simulink model "DUC"  (R2017b)
settings: Solver=VariableStepAuto  StartTime=0.0  StopTime=10.0  RelTol=1e-3
libraries: dspsigops x16, simulink x8
(part 2 of 2)

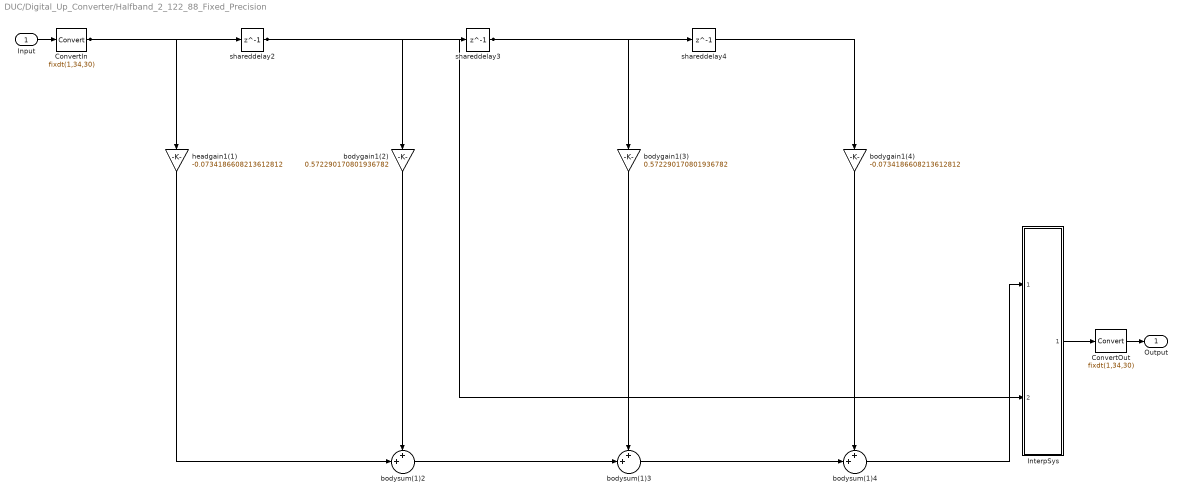
== system DUC/Digital_Up_Converter/Halfband_2_122_88_Fixed_Precision ==
  Input : Inport
  ConvertIn : DataTypeConversion  OutDataTypeStr=fixdt(1,34,30)  RndMeth=Nearest  SaturateOnIntegerOverflow=on
  ConvertOut : DataTypeConversion  OutDataTypeStr=fixdt(1,34,30)  SaturateOnIntegerOverflow=on
  InterpSys : Subsystem  Tag=FilterWizardInterpolatorCommutator
  bodygain1(2) : Gain  Gain=0.572290170801936782  ParamDataTypeStr=fixdt(1,36,34)  OutDataTypeStr=fixdt(1,36,32)  SaturateOnIntegerOverflow=on
  bodygain1(3) : Gain  Gain=0.572290170801936782  ParamDataTypeStr=fixdt(1,36,34)  OutDataTypeStr=fixdt(1,36,32)  SaturateOnIntegerOverflow=on
  bodygain1(4) : Gain  Gain=-0.0734186608213612812  ParamDataTypeStr=fixdt(1,36,34)  OutDataTypeStr=fixdt(1,36,32)  SaturateOnIntegerOverflow=on
  bodysum(1)2 : Sum  Inputs=++|  AccumDataTypeStr=fixdt(1,69,64)  OutDataTypeStr=fixdt(1,36,32)  SaturateOnIntegerOverflow=on
  bodysum(1)3 : Sum  Inputs=++|  AccumDataTypeStr=fixdt(1,69,64)  OutDataTypeStr=fixdt(1,36,32)  SaturateOnIntegerOverflow=on
  bodysum(1)4 : Sum  Inputs=++|  AccumDataTypeStr=fixdt(1,69,64)  OutDataTypeStr=fixdt(1,36,32)  SaturateOnIntegerOverflow=on
  headgain1(1) : Gain  Gain=-0.0734186608213612812  ParamDataTypeStr=fixdt(1,36,34)  OutDataTypeStr=fixdt(1,36,32)  SaturateOnIntegerOverflow=on
  shareddelay2 : Delay  DelayLength=1  InitialCondition=0
  shareddelay3 : Delay  DelayLength=1  InitialCondition=0
  shareddelay4 : Delay  DelayLength=1  InitialCondition=0
  Output : Outport
  wires:
  headgain1(1)/1 -> bodysum(1)2/2
  Input/1 -> ConvertIn/1
  ConvertIn/1 -> headgain1(1)/1, shareddelay2/1
  bodygain1(2)/1 -> bodysum(1)2/1
  bodysum(1)2/1 -> bodysum(1)3/2
  shareddelay2/1 -> bodygain1(2)/1, InterpSys/2(input2), shareddelay3/1
  bodygain1(3)/1 -> bodysum(1)3/1
  bodysum(1)3/1 -> bodysum(1)4/2
  shareddelay3/1 -> bodygain1(3)/1, shareddelay4/1
  bodygain1(4)/1 -> bodysum(1)4/1
  bodysum(1)4/1 -> InterpSys/1(input1)
  shareddelay4/1 -> bodygain1(4)/1
  InterpSys/1(output) -> ConvertOut/1
  ConvertOut/1 -> Output/1

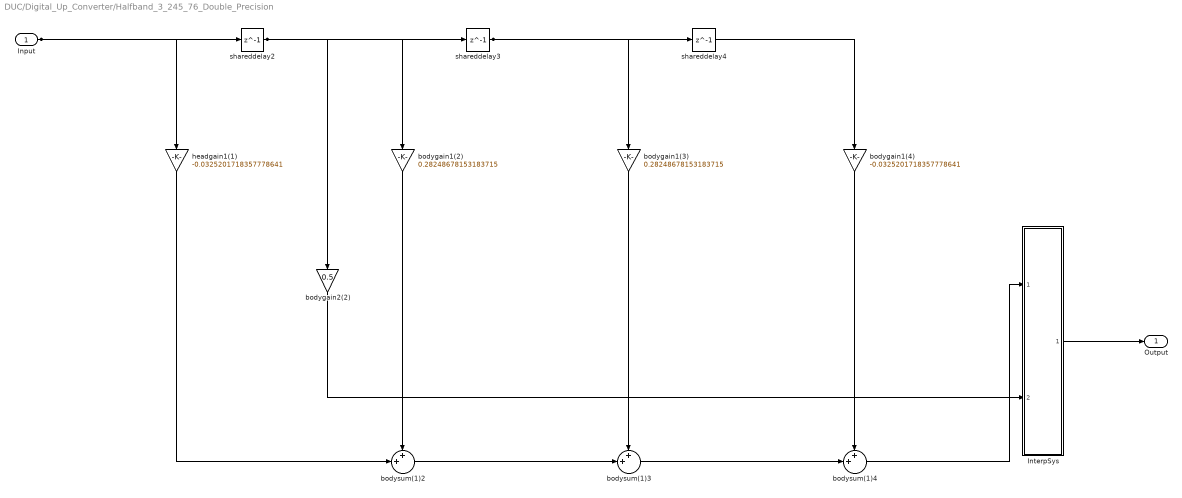
== system DUC/Digital_Up_Converter/Halfband_3_245_76_Double_Precision ==
  Input : Inport
  InterpSys : Subsystem  Tag=FilterWizardInterpolatorCommutator
  bodygain1(2) : Gain  Gain=0.28248678153183715  ParamDataTypeStr=double  RndMeth=Nearest  SaturateOnIntegerOverflow=on  OutDataTypeStr=Inherit: Same as input
  bodygain1(3) : Gain  Gain=0.28248678153183715  ParamDataTypeStr=double  RndMeth=Nearest  SaturateOnIntegerOverflow=on  OutDataTypeStr=Inherit: Same as input
  bodygain1(4) : Gain  Gain=-0.0325201718357778641  ParamDataTypeStr=double  RndMeth=Nearest  SaturateOnIntegerOverflow=on  OutDataTypeStr=Inherit: Same as input
  bodygain2(2) : Gain  Gain=0.5  ParamDataTypeStr=double  RndMeth=Nearest  SaturateOnIntegerOverflow=on  OutDataTypeStr=Inherit: Same as input
  bodysum(1)2 : Sum  Inputs=++|  RndMeth=Nearest  SaturateOnIntegerOverflow=on  OutDataTypeStr=Inherit: Same as first input
  bodysum(1)3 : Sum  Inputs=++|  RndMeth=Nearest  SaturateOnIntegerOverflow=on  OutDataTypeStr=Inherit: Same as first input
  bodysum(1)4 : Sum  Inputs=++|  RndMeth=Nearest  SaturateOnIntegerOverflow=on  OutDataTypeStr=Inherit: Same as first input
  headgain1(1) : Gain  Gain=-0.0325201718357778641  ParamDataTypeStr=double  RndMeth=Nearest  SaturateOnIntegerOverflow=on  OutDataTypeStr=Inherit: Same as input
  shareddelay2 : Delay  DelayLength=1  InitialCondition=0
  shareddelay3 : Delay  DelayLength=1  InitialCondition=0
  shareddelay4 : Delay  DelayLength=1  InitialCondition=0
  Output : Outport
  wires:
  headgain1(1)/1 -> bodysum(1)2/2
  Input/1 -> headgain1(1)/1, shareddelay2/1
  bodygain1(2)/1 -> bodysum(1)2/1
  bodygain2(2)/1 -> InterpSys/2(input2)
  bodysum(1)2/1 -> bodysum(1)3/2
  shareddelay2/1 -> bodygain1(2)/1, bodygain2(2)/1, shareddelay3/1
  bodygain1(3)/1 -> bodysum(1)3/1
  bodysum(1)3/1 -> bodysum(1)4/2
  shareddelay3/1 -> bodygain1(3)/1, shareddelay4/1
  bodygain1(4)/1 -> bodysum(1)4/1
  bodysum(1)4/1 -> InterpSys/1(input1)
  shareddelay4/1 -> bodygain1(4)/1
  InterpSys/1(output) -> Output/1

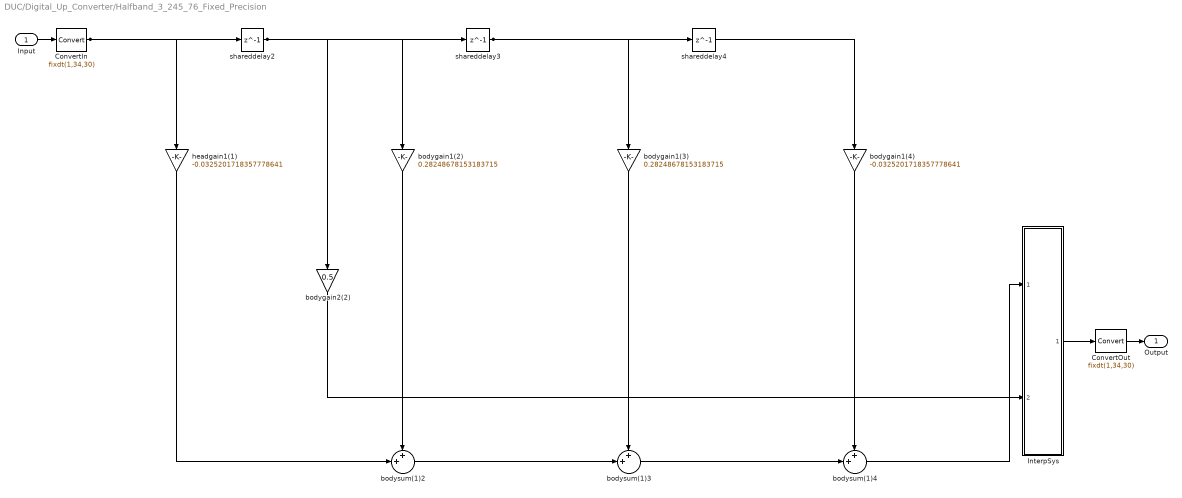
== system DUC/Digital_Up_Converter/Halfband_3_245_76_Fixed_Precision ==
  Input : Inport
  ConvertIn : DataTypeConversion  OutDataTypeStr=fixdt(1,34,30)  RndMeth=Nearest  SaturateOnIntegerOverflow=on
  ConvertOut : DataTypeConversion  OutDataTypeStr=fixdt(1,34,30)  SaturateOnIntegerOverflow=on
  InterpSys : Subsystem  Tag=FilterWizardInterpolatorCommutator
  bodygain1(2) : Gain  Gain=0.28248678153183715  ParamDataTypeStr=fixdt(1,36,35)  OutDataTypeStr=fixdt(1,36,32)  SaturateOnIntegerOverflow=on
  bodygain1(3) : Gain  Gain=0.28248678153183715  ParamDataTypeStr=fixdt(1,36,35)  OutDataTypeStr=fixdt(1,36,32)  SaturateOnIntegerOverflow=on
  bodygain1(4) : Gain  Gain=-0.0325201718357778641  ParamDataTypeStr=fixdt(1,36,35)  OutDataTypeStr=fixdt(1,36,32)  SaturateOnIntegerOverflow=on
  bodygain2(2) : Gain  Gain=0.5  ParamDataTypeStr=fixdt(1,36,35)  OutDataTypeStr=fixdt(1,36,32)  SaturateOnIntegerOverflow=on
  bodysum(1)2 : Sum  Inputs=++|  AccumDataTypeStr=fixdt(1,69,65)  OutDataTypeStr=fixdt(1,36,32)  SaturateOnIntegerOverflow=on
  bodysum(1)3 : Sum  Inputs=++|  AccumDataTypeStr=fixdt(1,69,65)  OutDataTypeStr=fixdt(1,36,32)  SaturateOnIntegerOverflow=on
  bodysum(1)4 : Sum  Inputs=++|  AccumDataTypeStr=fixdt(1,69,65)  OutDataTypeStr=fixdt(1,36,32)  SaturateOnIntegerOverflow=on
  headgain1(1) : Gain  Gain=-0.0325201718357778641  ParamDataTypeStr=fixdt(1,36,35)  OutDataTypeStr=fixdt(1,36,32)  SaturateOnIntegerOverflow=on
  shareddelay2 : Delay  DelayLength=1  InitialCondition=0
  shareddelay3 : Delay  DelayLength=1  InitialCondition=0
  shareddelay4 : Delay  DelayLength=1  InitialCondition=0
  Output : Outport
  wires:
  headgain1(1)/1 -> bodysum(1)2/2
  Input/1 -> ConvertIn/1
  ConvertIn/1 -> headgain1(1)/1, shareddelay2/1
  bodygain1(2)/1 -> bodysum(1)2/1
  bodygain2(2)/1 -> InterpSys/2(input2)
  bodysum(1)2/1 -> bodysum(1)3/2
  shareddelay2/1 -> bodygain1(2)/1, bodygain2(2)/1, shareddelay3/1
  bodygain1(3)/1 -> bodysum(1)3/1
  bodysum(1)3/1 -> bodysum(1)4/2
  shareddelay3/1 -> bodygain1(3)/1, shareddelay4/1
  bodygain1(4)/1 -> bodysum(1)4/1
  bodysum(1)4/1 -> InterpSys/1(input1)
  shareddelay4/1 -> bodygain1(4)/1
  InterpSys/1(output) -> ConvertOut/1
  ConvertOut/1 -> Output/1

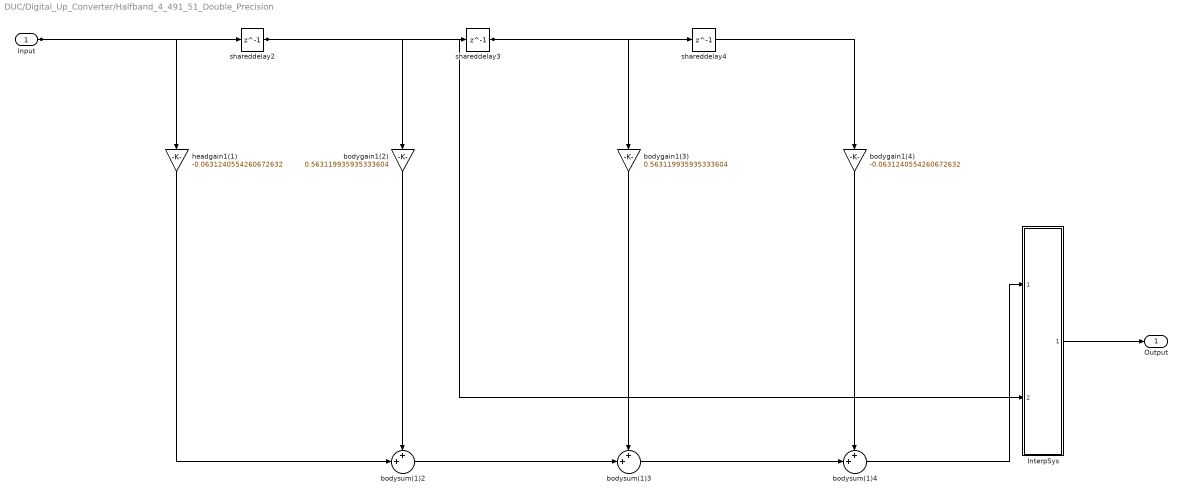
== system DUC/Digital_Up_Converter/Halfband_4_491_51_Double_Precision ==
  Input : Inport
  InterpSys : Subsystem  Tag=FilterWizardInterpolatorCommutator
  bodygain1(2) : Gain  Gain=0.563119935935333604  ParamDataTypeStr=double  RndMeth=Nearest  SaturateOnIntegerOverflow=on  OutDataTypeStr=Inherit: Same as input
  bodygain1(3) : Gain  Gain=0.563119935935333604  ParamDataTypeStr=double  RndMeth=Nearest  SaturateOnIntegerOverflow=on  OutDataTypeStr=Inherit: Same as input
  bodygain1(4) : Gain  Gain=-0.0631240554260672632  ParamDataTypeStr=double  RndMeth=Nearest  SaturateOnIntegerOverflow=on  OutDataTypeStr=Inherit: Same as input
  bodysum(1)2 : Sum  Inputs=++|  RndMeth=Nearest  SaturateOnIntegerOverflow=on  OutDataTypeStr=Inherit: Same as first input
  bodysum(1)3 : Sum  Inputs=++|  RndMeth=Nearest  SaturateOnIntegerOverflow=on  OutDataTypeStr=Inherit: Same as first input
  bodysum(1)4 : Sum  Inputs=++|  RndMeth=Nearest  SaturateOnIntegerOverflow=on  OutDataTypeStr=Inherit: Same as first input
  headgain1(1) : Gain  Gain=-0.0631240554260672632  ParamDataTypeStr=double  RndMeth=Nearest  SaturateOnIntegerOverflow=on  OutDataTypeStr=Inherit: Same as input
  shareddelay2 : Delay  DelayLength=1  InitialCondition=0
  shareddelay3 : Delay  DelayLength=1  InitialCondition=0
  shareddelay4 : Delay  DelayLength=1  InitialCondition=0
  Output : Outport
  wires:
  headgain1(1)/1 -> bodysum(1)2/2
  Input/1 -> headgain1(1)/1, shareddelay2/1
  bodygain1(2)/1 -> bodysum(1)2/1
  bodysum(1)2/1 -> bodysum(1)3/2
  shareddelay2/1 -> bodygain1(2)/1, InterpSys/2(input2), shareddelay3/1
  bodygain1(3)/1 -> bodysum(1)3/1
  bodysum(1)3/1 -> bodysum(1)4/2
  shareddelay3/1 -> bodygain1(3)/1, shareddelay4/1
  bodygain1(4)/1 -> bodysum(1)4/1
  bodysum(1)4/1 -> InterpSys/1(input1)
  shareddelay4/1 -> bodygain1(4)/1
  InterpSys/1(output) -> Output/1

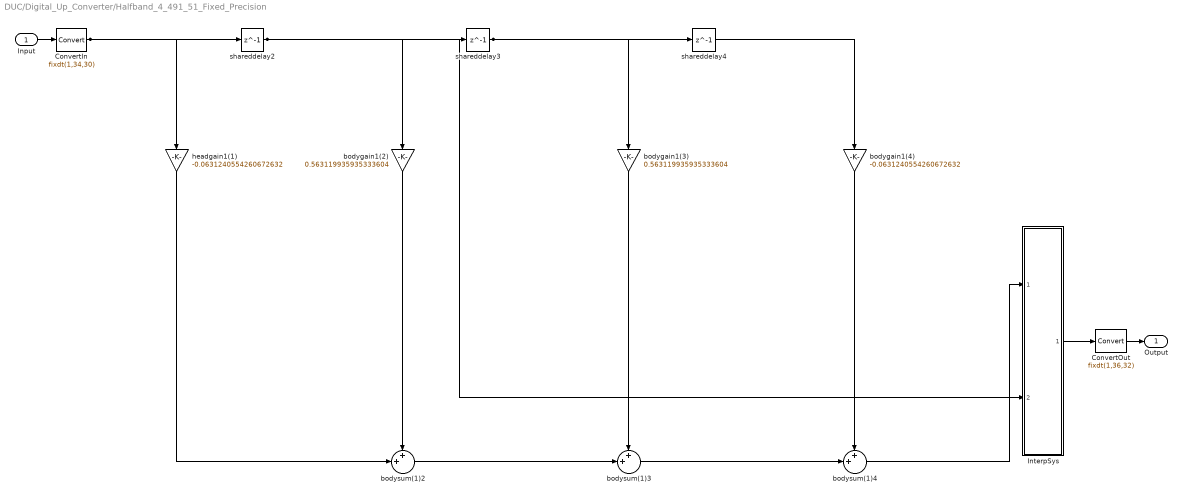
== system DUC/Digital_Up_Converter/Halfband_4_491_51_Fixed_Precision ==
  Input : Inport
  ConvertIn : DataTypeConversion  OutDataTypeStr=fixdt(1,34,30)  RndMeth=Nearest  SaturateOnIntegerOverflow=on
  ConvertOut : DataTypeConversion  OutDataTypeStr=fixdt(1,36,32)  SaturateOnIntegerOverflow=on
  InterpSys : Subsystem  Tag=FilterWizardInterpolatorCommutator
  bodygain1(2) : Gain  Gain=0.563119935935333604  ParamDataTypeStr=fixdt(1,36,34)  OutDataTypeStr=fixdt(1,36,32)  SaturateOnIntegerOverflow=on
  bodygain1(3) : Gain  Gain=0.563119935935333604  ParamDataTypeStr=fixdt(1,36,34)  OutDataTypeStr=fixdt(1,36,32)  SaturateOnIntegerOverflow=on
  bodygain1(4) : Gain  Gain=-0.0631240554260672632  ParamDataTypeStr=fixdt(1,36,34)  OutDataTypeStr=fixdt(1,36,32)  SaturateOnIntegerOverflow=on
  bodysum(1)2 : Sum  Inputs=++|  AccumDataTypeStr=fixdt(1,69,64)  OutDataTypeStr=fixdt(1,36,32)  SaturateOnIntegerOverflow=on
  bodysum(1)3 : Sum  Inputs=++|  AccumDataTypeStr=fixdt(1,69,64)  OutDataTypeStr=fixdt(1,36,32)  SaturateOnIntegerOverflow=on
  bodysum(1)4 : Sum  Inputs=++|  AccumDataTypeStr=fixdt(1,69,64)  OutDataTypeStr=fixdt(1,36,32)  SaturateOnIntegerOverflow=on
  headgain1(1) : Gain  Gain=-0.0631240554260672632  ParamDataTypeStr=fixdt(1,36,34)  OutDataTypeStr=fixdt(1,36,32)  SaturateOnIntegerOverflow=on
  shareddelay2 : Delay  DelayLength=1  InitialCondition=0
  shareddelay3 : Delay  DelayLength=1  InitialCondition=0
  shareddelay4 : Delay  DelayLength=1  InitialCondition=0
  Output : Outport
  wires:
  headgain1(1)/1 -> bodysum(1)2/2
  Input/1 -> ConvertIn/1
  ConvertIn/1 -> headgain1(1)/1, shareddelay2/1
  bodygain1(2)/1 -> bodysum(1)2/1
  bodysum(1)2/1 -> bodysum(1)3/2
  shareddelay2/1 -> bodygain1(2)/1, InterpSys/2(input2), shareddelay3/1
  bodygain1(3)/1 -> bodysum(1)3/1
  bodysum(1)3/1 -> bodysum(1)4/2
  shareddelay3/1 -> bodygain1(3)/1, shareddelay4/1
  bodygain1(4)/1 -> bodysum(1)4/1
  bodysum(1)4/1 -> InterpSys/1(input1)
  shareddelay4/1 -> bodygain1(4)/1
  InterpSys/1(output) -> ConvertOut/1
  ConvertOut/1 -> Output/1

== system DUC/Digital_Up_Converter/Halfband_1_61_44_Double_Precision/InterpSys ==
  input1 : Inport
  input2 : Inport  Port=2
  delay1 : Delay  DelayLength=1
  multiswitch : MultiPortSwitch  DataPortOrder=Zero-based contiguous  Inputs=2  zeroidx=on  SaturateOnIntegerOverflow=on
  ringcounter : simulink/Sources/Counter Limited  uplimit=1  tsamp=-1
  upsamp1 : dspsigops/Upsample  N=2  phase=0  RateOptions=Allow multirate processing  ic=0  mode=Unused parameter value
  upsamp2 : dspsigops/Upsample  N=2  phase=0  RateOptions=Allow multirate processing  ic=0  mode=Unused parameter value
  output : Outport
  wires:
  ringcounter/1 -> multiswitch/1
  input1/1 -> upsamp1/1
  upsamp1/1 -> multiswitch/2
  input2/1 -> upsamp2/1
  upsamp2/1 -> delay1/1
  delay1/1 -> multiswitch/3
  multiswitch/1 -> output/1

== system DUC/Digital_Up_Converter/Halfband_1_61_44_Fixed_Precision/InterpSys ==
  input1 : Inport
  input2 : Inport  Port=2
  delay1 : Delay  DelayLength=1
  multiswitch : MultiPortSwitch  DataPortOrder=Zero-based contiguous  Inputs=2  zeroidx=on  SaturateOnIntegerOverflow=on
  ringcounter : simulink/Sources/Counter Limited  uplimit=1  tsamp=-1
  upsamp1 : dspsigops/Upsample  N=2  phase=0  RateOptions=Allow multirate processing  ic=0  mode=Unused parameter value
  upsamp2 : dspsigops/Upsample  N=2  phase=0  RateOptions=Allow multirate processing  ic=0  mode=Unused parameter value
  output : Outport
  wires:
  ringcounter/1 -> multiswitch/1
  input1/1 -> upsamp1/1
  upsamp1/1 -> multiswitch/2
  input2/1 -> upsamp2/1
  upsamp2/1 -> delay1/1
  delay1/1 -> multiswitch/3
  multiswitch/1 -> output/1

== system DUC/Digital_Up_Converter/Halfband_2_122_88_Double_Precision/InterpSys ==
  input1 : Inport
  input2 : Inport  Port=2
  delay1 : Delay  DelayLength=1
  multiswitch : MultiPortSwitch  DataPortOrder=Zero-based contiguous  Inputs=2  zeroidx=on  SaturateOnIntegerOverflow=on
  ringcounter : simulink/Sources/Counter Limited  uplimit=1  tsamp=-1
  upsamp1 : dspsigops/Upsample  N=2  phase=0  RateOptions=Allow multirate processing  ic=0  mode=Unused parameter value
  upsamp2 : dspsigops/Upsample  N=2  phase=0  RateOptions=Allow multirate processing  ic=0  mode=Unused parameter value
  output : Outport
  wires:
  ringcounter/1 -> multiswitch/1
  input1/1 -> upsamp1/1
  upsamp1/1 -> multiswitch/2
  input2/1 -> upsamp2/1
  upsamp2/1 -> delay1/1
  delay1/1 -> multiswitch/3
  multiswitch/1 -> output/1

== system DUC/Digital_Up_Converter/Halfband_2_122_88_Fixed_Precision/InterpSys ==
  input1 : Inport
  input2 : Inport  Port=2
  delay1 : Delay  DelayLength=1
  multiswitch : MultiPortSwitch  DataPortOrder=Zero-based contiguous  Inputs=2  zeroidx=on  SaturateOnIntegerOverflow=on
  ringcounter : simulink/Sources/Counter Limited  uplimit=1  tsamp=-1
  upsamp1 : dspsigops/Upsample  N=2  phase=0  RateOptions=Allow multirate processing  ic=0  mode=Unused parameter value
  upsamp2 : dspsigops/Upsample  N=2  phase=0  RateOptions=Allow multirate processing  ic=0  mode=Unused parameter value
  output : Outport
  wires:
  ringcounter/1 -> multiswitch/1
  input1/1 -> upsamp1/1
  upsamp1/1 -> multiswitch/2
  input2/1 -> upsamp2/1
  upsamp2/1 -> delay1/1
  delay1/1 -> multiswitch/3
  multiswitch/1 -> output/1

== system DUC/Digital_Up_Converter/Halfband_3_245_76_Double_Precision/InterpSys ==
  input1 : Inport
  input2 : Inport  Port=2
  delay1 : Delay  DelayLength=1
  multiswitch : MultiPortSwitch  DataPortOrder=Zero-based contiguous  Inputs=2  zeroidx=on  SaturateOnIntegerOverflow=on
  ringcounter : simulink/Sources/Counter Limited  uplimit=1  tsamp=-1
  upsamp1 : dspsigops/Upsample  N=2  phase=0  RateOptions=Allow multirate processing  ic=0  mode=Unused parameter value
  upsamp2 : dspsigops/Upsample  N=2  phase=0  RateOptions=Allow multirate processing  ic=0  mode=Unused parameter value
  output : Outport
  wires:
  ringcounter/1 -> multiswitch/1
  input1/1 -> upsamp1/1
  upsamp1/1 -> multiswitch/2
  input2/1 -> upsamp2/1
  upsamp2/1 -> delay1/1
  delay1/1 -> multiswitch/3
  multiswitch/1 -> output/1

== system DUC/Digital_Up_Converter/Halfband_3_245_76_Fixed_Precision/InterpSys ==
  input1 : Inport
  input2 : Inport  Port=2
  delay1 : Delay  DelayLength=1
  multiswitch : MultiPortSwitch  DataPortOrder=Zero-based contiguous  Inputs=2  zeroidx=on  SaturateOnIntegerOverflow=on
  ringcounter : simulink/Sources/Counter Limited  uplimit=1  tsamp=-1
  upsamp1 : dspsigops/Upsample  N=2  phase=0  RateOptions=Allow multirate processing  ic=0  mode=Unused parameter value
  upsamp2 : dspsigops/Upsample  N=2  phase=0  RateOptions=Allow multirate processing  ic=0  mode=Unused parameter value
  output : Outport
  wires:
  ringcounter/1 -> multiswitch/1
  input1/1 -> upsamp1/1
  upsamp1/1 -> multiswitch/2
  input2/1 -> upsamp2/1
  upsamp2/1 -> delay1/1
  delay1/1 -> multiswitch/3
  multiswitch/1 -> output/1

== system DUC/Digital_Up_Converter/Halfband_4_491_51_Double_Precision/InterpSys ==
  input1 : Inport
  input2 : Inport  Port=2
  delay1 : Delay  DelayLength=1
  multiswitch : MultiPortSwitch  DataPortOrder=Zero-based contiguous  Inputs=2  zeroidx=on  SaturateOnIntegerOverflow=on
  ringcounter : simulink/Sources/Counter Limited  uplimit=1  tsamp=-1
  upsamp1 : dspsigops/Upsample  N=2  phase=0  RateOptions=Allow multirate processing  ic=0  mode=Unused parameter value
  upsamp2 : dspsigops/Upsample  N=2  phase=0  RateOptions=Allow multirate processing  ic=0  mode=Unused parameter value
  output : Outport
  wires:
  ringcounter/1 -> multiswitch/1
  input1/1 -> upsamp1/1
  upsamp1/1 -> multiswitch/2
  input2/1 -> upsamp2/1
  upsamp2/1 -> delay1/1
  delay1/1 -> multiswitch/3
  multiswitch/1 -> output/1

== system DUC/Digital_Up_Converter/Halfband_4_491_51_Fixed_Precision/InterpSys ==
  input1 : Inport
  input2 : Inport  Port=2
  delay1 : Delay  DelayLength=1
  multiswitch : MultiPortSwitch  DataPortOrder=Zero-based contiguous  Inputs=2  zeroidx=on  SaturateOnIntegerOverflow=on
  ringcounter : simulink/Sources/Counter Limited  uplimit=1  tsamp=-1
  upsamp1 : dspsigops/Upsample  N=2  phase=0  RateOptions=Allow multirate processing  ic=0  mode=Unused parameter value
  upsamp2 : dspsigops/Upsample  N=2  phase=0  RateOptions=Allow multirate processing  ic=0  mode=Unused parameter value
  output : Outport
  wires:
  ringcounter/1 -> multiswitch/1
  input1/1 -> upsamp1/1
  upsamp1/1 -> multiswitch/2
  input2/1 -> upsamp2/1
  upsamp2/1 -> delay1/1
  delay1/1 -> multiswitch/3
  multiswitch/1 -> output/1
